simulink model "x1_Pn_sequence"  (R2023b)
settings: Solver=FixedStepDiscrete  StartTime=0.0  StopTime=62  RelTol=1e-3
PreLoadFcn:
  | iniStates = [ 0 0 1 0 1 1];
libraries: commseqgen3 x1
settings Model: Creator=The MathWorks, Inc.  LastModifiedBy=Abhi Singh
settings SolverCC: AlgebraicLoopSolver=TrustRegion
settings DataIOCC: LimitDataPoints=on  SaveFormat=Array  ReturnWorkspaceOutputs=off
settings OptimizationCC: ExpressionDepthLimit=2147483647  InitFltsAndDblsToZero=on  LifeSpan=1  EfficientTunableParamExpr=on
settings DebuggingCC: SaveWithParameterizedLinksMsg=none  UnderspecifiedInitializationDetection=Classic  MergeDetectMultiDrivingBlocksExec=none  SignalResolutionControl=TryResolveAllWithWarning  SolverPrmCheckMsg=warning  MultiTaskDSMMsg=warning  MultiTaskCondExecSysMsg=none  FcnCallInpInsideContextMsg=warning  UnconnectedInputMsg=warning  UnconnectedOutputMsg=warning  UnconnectedLineMsg=warning  AllowSymbolicDim=off  StateNameClashWarn=warning  SFUnexpectedBacktrackingDiag=warning  SFNoUnconditionalDefaultTransitionDiag=warning  SFExecutionAtInitializationDiag=none  ArithmeticOperatorsInVariantConditions=warning
settings HardwareCC: ProdBitPerPointer=32  ProdBitPerSizeT=32  ProdBitPerPtrDiffT=32  ProdLargestAtomicFloat=None  ProdIntDivRoundTo=Undefined  ProdEndianess=Unspecified  ProdWordSize=32  ProdHWDeviceType=32-bit Generic
settings ModelReferenceCC: EnableRefExpFcnMdlSchedulingChecks=on  PropagateSignalLabelsOutOfModel=off
settings SFSimCC: SimUseLocalCustomCode=off  MATLABDynamicMemAlloc=off  CustomCodeUndefinedFunction=UseInterfaceOnly
settings RTWCC: Description=Real-Time Workshop Embedded Coder (no auto configuration)  SystemTargetFile=ert.tlc  GenCodeOnly=on  TemplateMakefile=ert_default_tmf  RTWUseLocalCustomCode=off
settings CodeAppCC: IgnoreCustomStorageClasses=off  CustomSymbolStrType=$N$R$M  StateflowObjectComments=on  InternalIdentifier=Classic
settings ERTTargetCC: TargetFcnLib=ansi_tfl_tmw.mat  MultiwordLength=2048  GenerateSampleERTMain=on  ERTCustomFileTemplate=example_file_process.tlc  ConvertIfToSwitch=off  SuppressUnreachableDefaultCases=off
settings ConfigComp: CovMetricSettings=dw  CovSaveCumulativeToWorkspaceVar=on  CovSaveSingleToWorkspaceVar=on  CovExternalEMLEnable=off

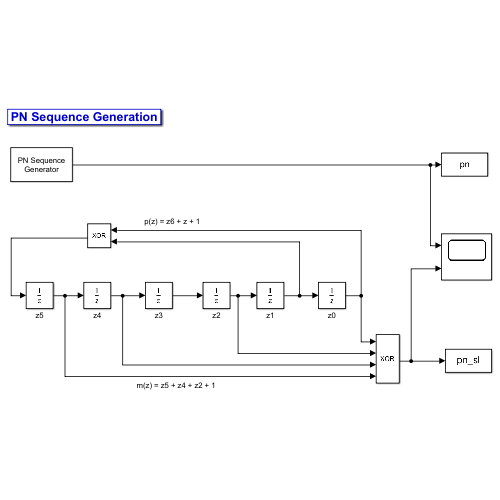
[thumbnail: Simulink's stored preview of the top-level diagram]
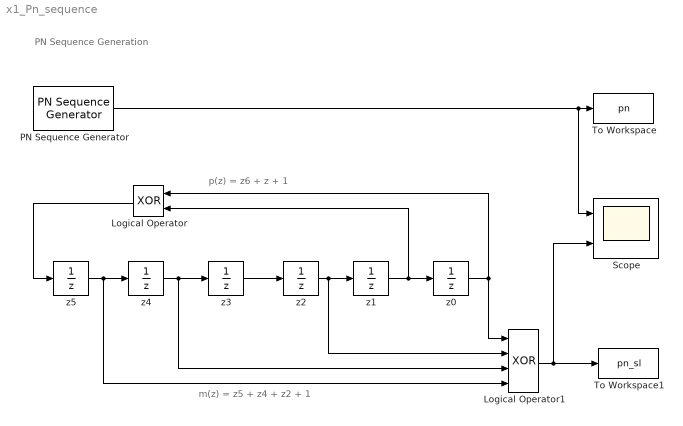
== system x1_Pn_sequence ==
  note: PN Sequence Generation
  note: p(z) = z6 + z + 1
  note: m(z) = z5 + z4 + z2 + 1
  Logical Operator : Logic  Operator=XOR  AllPortsSameDT=off  OutDataTypeStr=boolean
  Logical Operator1 : Logic  Operator=XOR  Inputs=4  AllPortsSameDT=off  OutDataTypeStr=boolean
  PN Sequence Generator : commseqgen3/PN Sequence Generator  poly=[1 0 0 0 0 1 1]  ini_sta=iniStates  outBitMaskSource=Dialog parameter  shift=[1 1 0 1 0 1]  outVarSiz=off  maxOutSizeMode=Dialog parameter  maxOutSize=[10 1]  Ts=1  sampPerFrame=1  reset=off  bitPackedOutputs=off  outDataType=boolean  numPackedBits=8  bitPackDataSigned=off  bitPackedOutDType=double
  Scope : Scope  NumInputPorts=2
  To Workspace : ToWorkspace  VariableName=pn  SampleTime=-1
      settings: Save2DSignal=2-D array (concatenate along first dimension)
  To Workspace1 : ToWorkspace  VariableName=pn_sl  SampleTime=-1
      settings: Save2DSignal=2-D array (concatenate along first dimension)
  z0 : UnitDelay  InitialCondition=iniStates(6)  SampleTime=-1  HasFrameUpgradeWarning=on
  z1 : UnitDelay  InitialCondition=iniStates(5)  SampleTime=-1  HasFrameUpgradeWarning=on
  z2 : UnitDelay  InitialCondition=iniStates(4)  SampleTime=-1  HasFrameUpgradeWarning=on
  z3 : UnitDelay  InitialCondition=iniStates(3)  SampleTime=-1  HasFrameUpgradeWarning=on
  z4 : UnitDelay  InitialCondition=iniStates(2)  SampleTime=-1  HasFrameUpgradeWarning=on
  z5 : UnitDelay  InitialCondition=iniStates(1)  SampleTime=-1  HasFrameUpgradeWarning=on
  wires:
  Logical Operator/1 -> z5/1
  z5/1 -> z4/1, Logical Operator1/4
  z4/1 -> z3/1, Logical Operator1/3
  z3/1 -> z2/1
  z2/1 -> z1/1, Logical Operator1/2
  z1/1 -> z0/1, Logical Operator/2
  z0/1 -> Logical Operator1/1, Logical Operator/1
  Logical Operator1/1 -> Scope/2, To Workspace1/1
  PN Sequence Generator/1 -> Scope/1, To Workspace/1
